simulink model "non_linear_model"  (R2021b)
settings: Solver=VariableStepAuto  StartTime=0.0  StopTime=10.0  RelTol=1e-3
settings Model: Creator=varunsampat  LastModifiedBy=varunsampat

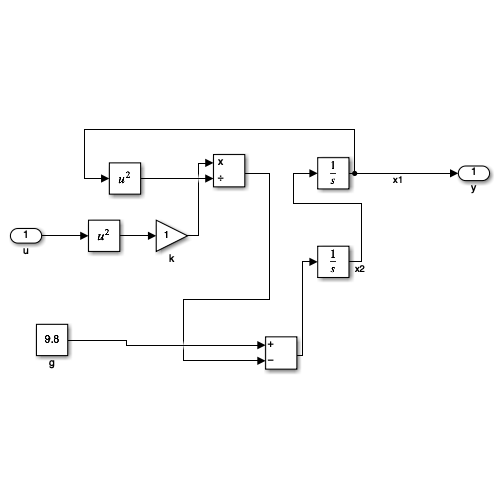
[thumbnail: Simulink's stored preview of the top-level diagram]
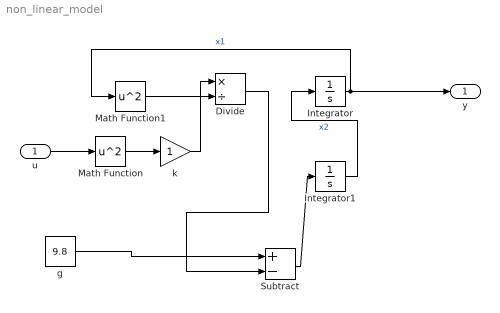
== system non_linear_model ==
  u : Inport
  Divide : Product  Inputs=*/
  Integrator : Integrator
  Integrator1 : Integrator
  Math Function : Math  Operator=square  SaturateOnIntegerOverflow=on
  Math Function1 : Math  Operator=square  SaturateOnIntegerOverflow=on
  Subtract : Sum  Inputs=+-
  g : Constant  Value=9.8
  k : Gain
  y : Outport
  wires:
  Integrator/1 -> Math Function1/1, y/1  "x1"
  u/1 -> Math Function/1
  Integrator1/1 -> Integrator/1  "x2"
  Math Function/1 -> k/1
  k/1 -> Divide/1
  Math Function1/1 -> Divide/2
  Divide/1 -> Subtract/2
  g/1 -> Subtract/1
  Subtract/1 -> Integrator1/1
